simulink model "simulink_interface"  (R2015a)
settings: Solver=ode45  StartTime=0.0  StopTime=inf  RelTol=1e-3
libraries: etargetslib x7, dspbuff3 x3, instrumentlib x3, dspnetwork x3, simulink x1
settings Model: Creator=zev  LastModifiedBy=zev

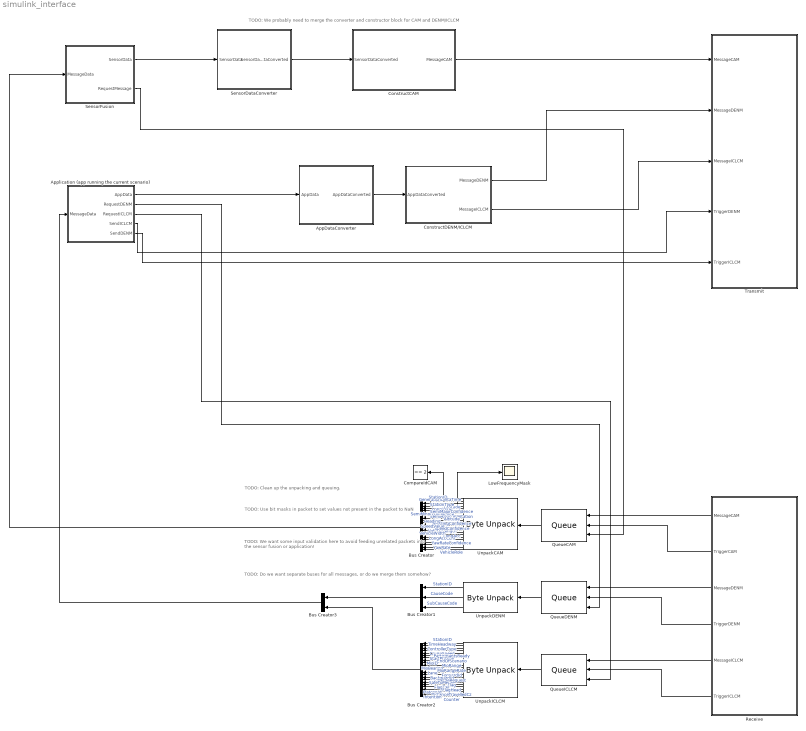
== system simulink_interface ==
  note: TODO: Clean up the unpacking and queuing.
  note: TODO: Do we want separate buses for all messages, or do we merge them somehow?
  note: TODO: Use bit masks in packet to set values not present in the packet to NaN
  note: TODO: We probably need to merge the converter and constructor block for CAM and DENM/ICLCM
  note: TODO: We want some input validation here to avoid feeding unrelated packets
      | into the sensor fusion or application!
  AppDataConverter : Subsystem
  Application (app running the current scenario) : Subsystem
  Bus Creator : BusCreator  Inputs=20
  Bus Creator1 : BusCreator  Inputs=3
  Bus Creator2 : BusCreator  Inputs=23
  Bus Creator3 : BusCreator  Inputs=2
  CompareIdCAM : simulink/Logic and Bit Operations/Compare To Constant  relop===  const=2  OutDataTypeStr=uint8
  ConstructCAM : Subsystem
  ConstructDENM/ICLCM : Subsystem
  LowFrequencyMask : Scope
  QueueCAM : dspbuff3/Queue  depth=8  trigger=Rising edge  overflow=Dynamic reallocation  pes=Warning  eso=off  fso=off  nso=off  clr=off  clrOutport=off  adf=on
  QueueDENM : dspbuff3/Queue  depth=8  trigger=Rising edge  overflow=Dynamic reallocation  pes=Warning  eso=off  fso=off  nso=off  clr=off  clrOutport=off  adf=on
  QueueICLCM : dspbuff3/Queue  depth=8  trigger=Rising edge  overflow=Dynamic reallocation  pes=Warning  eso=off  fso=off  nso=off  clr=off  clrOutport=off  adf=on
  Receive : Subsystem
  SensorDataConverter : Subsystem
  SensorFusion : Subsystem
  Transmit : Subsystem
  UnpackCAM : etargetslib/Byte Unpack  dimensions={[1],[1],[1],[1],[1],[1],[1],[1],[1],[1],[1],[1],[1],[1],[1],[1],[1],[1],[1],[1],[1],[1],}  datatypes={'uint8','int32', 'int32','uint8','int32', 'int32','int32', 'int32','int32', 'int32','int32', 'int32','int32', 'int32','int32', 'int32','int32', 'int32','int32', 'int32','int32', 'int32',}  byteAlign=1
  UnpackDENM : etargetslib/Byte Unpack  dimensions={[1], [1], [1]}  datatypes={'int32', 'int32', 'int32'}  byteAlign=1
  UnpackICLCM : etargetslib/Byte Unpack  dimensions={[1],[1], [1],[1], [1],[1], [1],[1], [1],[1], [1],[1], [1],[1], [1],[1], [1],[1],[1],[1], [1],[1], [1]}  datatypes={'int32','int32', 'int32','int32', 'int32','int32', 'int32','int32', 'int32','int32', 'int32','int32', 'int32','int32', 'int32','int32', 'int32','int32', 'int32','int32', 'int32','int32', 'int32'}  byteAlign=1
  wires:
  UnpackCAM/1 -> CompareIdCAM/1
  UnpackCAM/4 -> LowFrequencyMask/1
  UnpackCAM/22 -> Bus Creator/20  "VehicleRole"
  UnpackCAM/21 -> Bus Creator/19  "YawRateConfidence"
  UnpackCAM/20 -> Bus Creator/18  "YawRate"
  UnpackCAM/19 -> Bus Creator/17  "LongAccConf"
  UnpackCAM/18 -> Bus Creator/16  "LongAcc"
  UnpackCAM/16 -> Bus Creator/14  "VehicleLength"
  UnpackCAM/17 -> Bus Creator/15  "VehicleWidth"
  UnpackCAM/15 -> Bus Creator/13  "SpeedConfidence"
  UnpackCAM/13 -> Bus Creator/11  "HeadingConfidence"
  UnpackCAM/14 -> Bus Creator/12  "SpeedValue"
  UnpackCAM/12 -> Bus Creator/10  "Heading"
  UnpackCAM/10 -> Bus Creator/8  "SemiMajorOrientation"
  UnpackCAM/11 -> Bus Creator/9  "Altitude"
  UnpackCAM/9 -> Bus Creator/7  "SemiMinorConfidence"
  UnpackCAM/7 -> Bus Creator/5  "Longitude"
  UnpackCAM/8 -> Bus Creator/6  "SemiMajorConfidence"
  UnpackCAM/6 -> Bus Creator/4  "Latitude"
  UnpackCAM/5 -> Bus Creator/3  "StationType"
  UnpackCAM/3 -> Bus Creator/2  "GenerationDeltaTime"
  UnpackCAM/2 -> Bus Creator/1  "StationID"
  Bus Creator/1 -> SensorFusion/1(MessageData)
  SensorFusion/2(RequestMessage) -> QueueCAM/3
  QueueCAM/1 -> UnpackCAM/1
  Application (app running the current scenario)/2(RequestDENM) -> QueueDENM/3
  Application (app running the current scenario)/3(RequestICLCM) -> QueueICLCM/3
  QueueDENM/1 -> UnpackDENM/1
  QueueICLCM/1 -> UnpackICLCM/1
  Application (app running the current scenario)/1(AppData) -> AppDataConverter/1(AppData)
  AppDataConverter/1(AppDataConverted) -> ConstructDENM/ICLCM/1(AppDataConverted)
  SensorFusion/1(SensorData) -> SensorDataConverter/1(SensorData)
  SensorDataConverter/1(SensorDataConverted) -> ConstructCAM/1(SensorDataConverted)
  UnpackICLCM/1 -> Bus Creator2/1  "StationID"
  UnpackICLCM/2 -> Bus Creator2/2  "ControllerType"
  UnpackICLCM/3 -> Bus Creator2/3  "TimeHeadway"
  UnpackICLCM/4 -> Bus Creator2/4  "CruiseSpeed"
  UnpackICLCM/5 -> Bus Creator2/5  "ParticipantsReady"
  UnpackICLCM/6 -> Bus Creator2/6  "StartPlatoon"
  UnpackICLCM/7 -> Bus Creator2/7  "EndOfScenario"
  UnpackICLCM/8 -> Bus Creator2/8  "MioID"
  UnpackICLCM/9 -> Bus Creator2/9  "MioRange"
  UnpackICLCM/10 -> Bus Creator2/10  "MioBearing"
  UnpackICLCM/11 -> Bus Creator2/11  "MioRangeRate"
  UnpackICLCM/12 -> Bus Creator2/12  "Lane"
  UnpackICLCM/13 -> Bus Creator2/13  "ForwardId"
  UnpackICLCM/14 -> Bus Creator2/14  "BackwardId"
  UnpackICLCM/15 -> Bus Creator2/15  "MergeRequest"
  UnpackICLCM/16 -> Bus Creator2/16  "SafeToMerge"
  UnpackICLCM/17 -> Bus Creator2/17  "Flag"
  UnpackICLCM/18 -> Bus Creator2/18  "FlagTail"
  UnpackICLCM/19 -> Bus Creator2/19  "FlagHead"
  UnpackICLCM/20 -> Bus Creator2/20  "PlatoonId"
  UnpackICLCM/21 -> Bus Creator2/21  "DistanceTravelledCz"
  UnpackICLCM/22 -> Bus Creator2/22  "Intention"
  Bus Creator1/1 -> Bus Creator3/1
  Bus Creator2/1 -> Bus Creator3/2
  UnpackICLCM/23 -> Bus Creator2/23  "Counter"
  UnpackDENM/1 -> Bus Creator1/1  "StationID"
  UnpackDENM/2 -> Bus Creator1/2  "CauseCode"
  UnpackDENM/3 -> Bus Creator1/3  "SubCauseCode"
  Bus Creator3/1 -> Application (app running the current scenario)/1(MessageData)
  ConstructCAM/1(MessageCAM) -> Transmit/1(MessageCAM)
  ConstructDENM/ICLCM/1(MessageDENM) -> Transmit/2(MessageDENM)
  ConstructDENM/ICLCM/2(MessageICLCM) -> Transmit/3(MessageICLCM)
  Application (app running the current scenario)/4(SendICLCM) -> Transmit/4(TriggerDENM)
  Application (app running the current scenario)/5(SendDENM) -> Transmit/5(TriggerICLCM)
  Receive/1(MessageCAM) -> QueueCAM/1
  Receive/2(TriggerCAM) -> QueueCAM/2
  Receive/3(MessageDENM) -> QueueDENM/1
  Receive/4(TriggerDENM) -> QueueDENM/2
  Receive/5(MessageICLCM) -> QueueICLCM/1
  Receive/6(TriggerICLCM) -> QueueICLCM/2

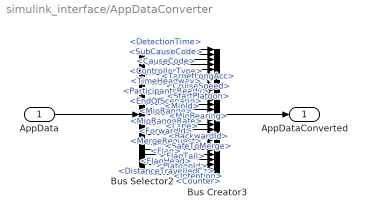
== system simulink_interface/AppDataConverter ==
  AppData : Inport
  Bus Creator3 : BusCreator  Inputs=26
  Bus Selector2 : BusSelector  OutputSignals=DetectionTime,CauseCode,SubCauseCode,ControllerType,TargetLongAcc,TimeHeadway,CruiseSpeed,ParticipantsReady,StartPlatoon,EndOfScenario,MioId,MioRange,MioBearing,MioRangeRate,Lane,ForwardId,BackwardId,MergeRequest,SafeToMerge,Flag,FlagTail,FlagHead,PlatoonId,DistanceTravelledCz,Intention,Counter
  AppDataConverted : Outport
  wires:
  Bus Creator3/1 -> AppDataConverted/1
  AppData/1 -> Bus Selector2/1
  Bus Selector2/1 -> Bus Creator3/1  "<DetectionTime>"
  Bus Selector2/2 -> Bus Creator3/2  "<CauseCode>"
  Bus Selector2/3 -> Bus Creator3/3  "<SubCauseCode>"
  Bus Selector2/4 -> Bus Creator3/4  "<ControllerType>"
  Bus Selector2/5 -> Bus Creator3/5  "<TargetLongAcc>"
  Bus Selector2/6 -> Bus Creator3/6  "<TimeHeadway>"
  Bus Selector2/7 -> Bus Creator3/7  "<CruiseSpeed>"
  Bus Selector2/8 -> Bus Creator3/8  "<ParticipantsReady>"
  Bus Selector2/9 -> Bus Creator3/9  "<StartPlatoon>"
  Bus Selector2/10 -> Bus Creator3/10  "<EndOfScenario>"
  Bus Selector2/11 -> Bus Creator3/11  "<MioId>"
  Bus Selector2/12 -> Bus Creator3/12  "<MioRange>"
  Bus Selector2/13 -> Bus Creator3/13  "<MioBearing>"
  Bus Selector2/14 -> Bus Creator3/14  "<MioRangeRate>"
  Bus Selector2/15 -> Bus Creator3/15  "<Lane>"
  Bus Selector2/16 -> Bus Creator3/16  "<ForwardId>"
  Bus Selector2/17 -> Bus Creator3/17  "<BackwardId>"
  Bus Selector2/18 -> Bus Creator3/18  "<MergeRequest>"
  Bus Selector2/19 -> Bus Creator3/19  "<SafeToMerge>"
  Bus Selector2/20 -> Bus Creator3/20  "<Flag>"
  Bus Selector2/21 -> Bus Creator3/21  "<FlagTail>"
  Bus Selector2/22 -> Bus Creator3/22  "<FlagHead>"
  Bus Selector2/23 -> Bus Creator3/23  "<PlatoonId>"
  Bus Selector2/24 -> Bus Creator3/24  "<DistanceTravelledCz>"
  Bus Selector2/25 -> Bus Creator3/25  "<Intention>"
  Bus Selector2/26 -> Bus Creator3/26  "<Counter>"

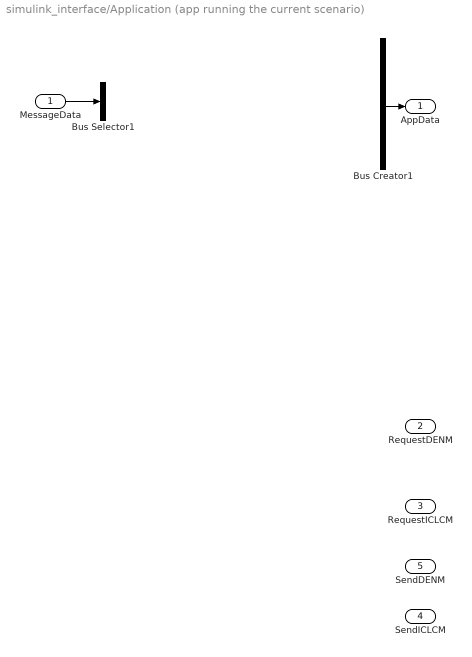
== system simulink_interface/Application (app running the current scenario) ==
  MessageData : Inport
  Bus Creator1 : BusCreator  Inputs=26
  Bus Selector1 : BusSelector  OutputSignals=signal1,signal2
  AppData : Outport
  RequestDENM : Outport  Port=2
  RequestICLCM : Outport  Port=3
  SendICLCM : Outport  Port=4
  SendDENM : Outport  Port=5
  wires:
  MessageData/1 -> Bus Selector1/1
  Bus Creator1/1 -> AppData/1
  ? -> Bus Creator1/1  "DetectionTime"
  ? -> Bus Creator1/2  "CauseCode"
  ? -> Bus Creator1/3  "SubCauseCode"
  ? -> Bus Creator1/4  "ControllerType"
  ? -> Bus Creator1/5  "TargetLongAcc"
  ? -> Bus Creator1/6  "TimeHeadway"
  ? -> Bus Creator1/7  "CruiseSpeed"
  ? -> Bus Creator1/8  "ParticipantsReady"
  ? -> Bus Creator1/9  "StartPlatoon"
  ? -> Bus Creator1/10  "EndOfScenario"
  ? -> Bus Creator1/11  "MioId"
  ? -> Bus Creator1/12  "MioRange"
  ? -> Bus Creator1/13  "MioBearing"
  ? -> Bus Creator1/14  "MioRangeRate"
  ? -> Bus Creator1/15  "Lane"
  ? -> Bus Creator1/16  "ForwardId"
  ? -> Bus Creator1/17  "BackwardId"
  ? -> Bus Creator1/18  "MergeRequest"
  ? -> Bus Creator1/19  "SafeToMerge"
  ? -> Bus Creator1/20  "Flag"
  ? -> Bus Creator1/21  "FlagTail"
  ? -> Bus Creator1/22  "FlagHead"
  ? -> Bus Creator1/23  "PlatoonId"
  ? -> Bus Creator1/24  "DistanceTravelledCz"
  ? -> Bus Creator1/25  "Intention"
  ? -> Bus Creator1/26  "Counter"

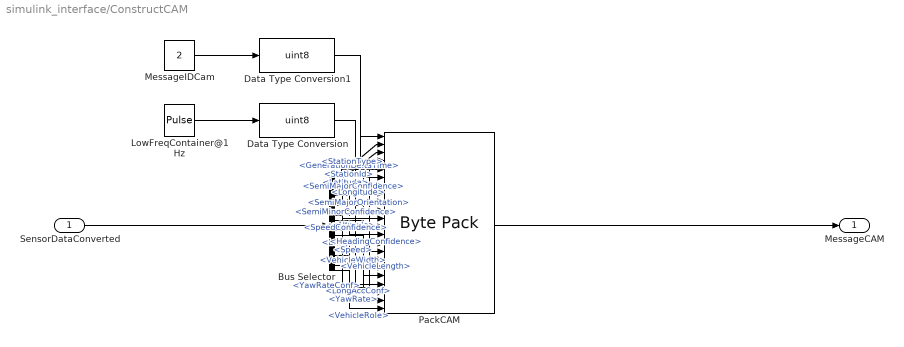
== system simulink_interface/ConstructCAM ==
  SensorDataConverted : Inport
  Bus Selector : BusSelector  OutputSignals=StationId,GenerationDeltaTime,StationType,Latitude,Longitude,SemiMajorConfidence,SemiMinorConfidence,SemiMajorOrientation,Altitude,Heading,HeadingConfidence,Speed,SpeedConfidence,VehicleLength,VehicleWidth,LongAcc,LongAccConf,YawRate,YawRateConf,VehicleRole
  Data Type Conversion : DataTypeConversion  OutDataTypeStr=uint8
  Data Type Conversion1 : DataTypeConversion  OutDataTypeStr=uint8
  LowFreqContainer@1Hz : DiscretePulseGenerator  PulseType=Time based  Amplitude=128  Period=1  PulseWidth=0.04
  MessageIDCam : Constant  Value=2
  PackCAM : etargetslib/Byte Pack  datatypes={'uint8','int32', 'int32','uint8','int32', 'int32','int32', 'int32','int32', 'int32','int32', 'int32','int32', 'int32','int32', 'int32','int32', 'int32','int32', 'int32','int32', 'int32',}  byteAlign=1
  MessageCAM : Outport
  wires:
  Bus Selector/8 -> PackCAM/10  "<SemiMajorOrientation>"
  Bus Selector/4 -> PackCAM/6  "<Latitude>"
  Bus Selector/2 -> PackCAM/3  "<GenerationDeltaTime>"
  Bus Selector/9 -> PackCAM/11  "<Altitude>"
  Bus Selector/6 -> PackCAM/8  "<SemiMajorConfidence>"
  Bus Selector/7 -> PackCAM/9  "<SemiMinorConfidence>"
  Bus Selector/1 -> PackCAM/2  "<StationId>"
  PackCAM/1 -> MessageCAM/1
  Bus Selector/3 -> PackCAM/5  "<StationType>"
  Data Type Conversion/1 -> PackCAM/4
  MessageIDCam/1 -> Data Type Conversion1/1
  Bus Selector/5 -> PackCAM/7  "<Longitude>"
  Bus Selector/15 -> PackCAM/17  "<VehicleWidth>"
  Bus Selector/10 -> PackCAM/12  "<Heading>"
  Bus Selector/16 -> PackCAM/18  "<LongAcc>"
  Bus Selector/12 -> PackCAM/14  "<Speed>"
  Bus Selector/17 -> PackCAM/19  "<LongAccConf>"
  Bus Selector/11 -> PackCAM/13  "<HeadingConfidence>"
  Bus Selector/14 -> PackCAM/16  "<VehicleLength>"
  Bus Selector/13 -> PackCAM/15  "<SpeedConfidence>"
  SensorDataConverted/1 -> Bus Selector/1
  Data Type Conversion1/1 -> PackCAM/1
  Bus Selector/19 -> PackCAM/21  "<YawRateConf>"
  Bus Selector/20 -> PackCAM/22  "<VehicleRole>"
  LowFreqContainer@1Hz/1 -> Data Type Conversion/1
  Bus Selector/18 -> PackCAM/20  "<YawRate>"

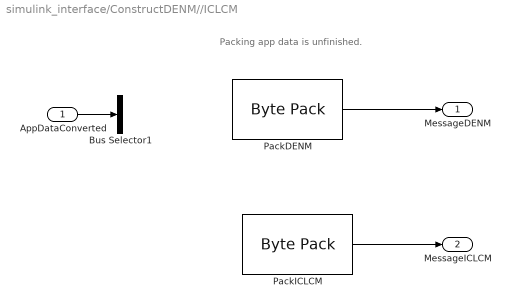
== system simulink_interface/ConstructDENM//ICLCM ==
  note: Packing app data is unfinished.
  AppDataConverted : Inport
  Bus Selector1 : BusSelector  OutputSignals=signal1,signal2
  PackDENM : etargetslib/Byte Pack  datatypes={'int32', 'int32'}  byteAlign=1
  PackICLCM : etargetslib/Byte Pack  datatypes={'int32', 'int32'}  byteAlign=1
  MessageDENM : Outport
  MessageICLCM : Outport  Port=2
  wires:
  PackDENM/1 -> MessageDENM/1
  AppDataConverted/1 -> Bus Selector1/1
  PackICLCM/1 -> MessageICLCM/1

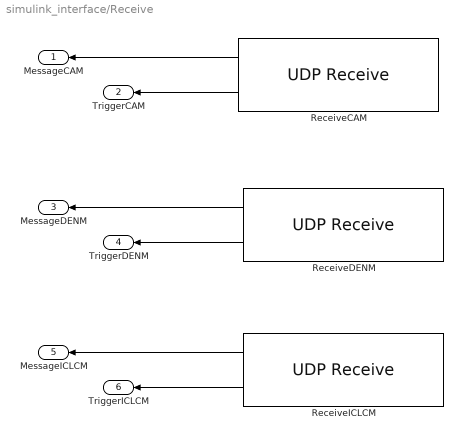
== system simulink_interface/Receive ==
  ReceiveCAM : instrumentlib/UDP Receive  Host=0.0.0.0  Port=5000  LocalPort=-1  DataSize="[1  82]"  EnableBlockingMode=off  Timeout=10  SampleTime=0.01  DataType=uint8  ByteOrder=BigEndian
  ReceiveDENM : instrumentlib/UDP Receive  Host=0.0.0.0  Port=5000  LocalPort=-1  DataSize="[1  82]"  EnableBlockingMode=off  Timeout=10  SampleTime=0.01  DataType=uint8  ByteOrder=BigEndian
  ReceiveICLCM : instrumentlib/UDP Receive  Host=0.0.0.0  Port=5000  LocalPort=-1  DataSize="[1  82]"  EnableBlockingMode=off  Timeout=10  SampleTime=0.01  DataType=uint8  ByteOrder=BigEndian
  MessageCAM : Outport
  TriggerCAM : Outport  Port=2
  MessageDENM : Outport  Port=3
  TriggerDENM : Outport  Port=4
  MessageICLCM : Outport  Port=5
  TriggerICLCM : Outport  Port=6
  wires:
  ReceiveCAM/1 -> MessageCAM/1
  ReceiveICLCM/2 -> TriggerICLCM/1
  ReceiveICLCM/1 -> MessageICLCM/1
  ReceiveDENM/2 -> TriggerDENM/1
  ReceiveDENM/1 -> MessageDENM/1
  ReceiveCAM/2 -> TriggerCAM/1

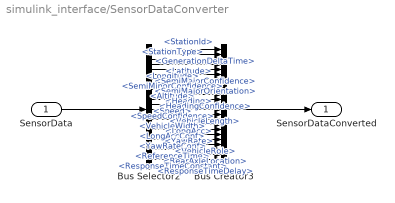
== system simulink_interface/SensorDataConverter ==
  SensorData : Inport
  Bus Creator3 : BusCreator  Inputs=24
  Bus Selector2 : BusSelector  OutputSignals=StationId,GenerationDeltaTime,StationType,Latitude,Longitude,SemiMajorConfidence,SemiMinorConfidence,SemiMajorOrientation,Altitude,Heading,HeadingConfidence,Speed,SpeedConfidence,VehicleLength,VehicleWidth,LongAcc,LongAccConf,YawRate,YawRateConf,VehicleRole,ReferenceTime,RearAxleLocation,ResponseTimeConstant,ResponseTimeDelay
  SensorDataConverted : Outport
  wires:
  Bus Creator3/1 -> SensorDataConverted/1
  SensorData/1 -> Bus Selector2/1
  Bus Selector2/1 -> Bus Creator3/1  "<StationId>"
  Bus Selector2/2 -> Bus Creator3/2  "<GenerationDeltaTime>"
  Bus Selector2/3 -> Bus Creator3/3  "<StationType>"
  Bus Selector2/4 -> Bus Creator3/4  "<Latitude>"
  Bus Selector2/5 -> Bus Creator3/5  "<Longitude>"
  Bus Selector2/6 -> Bus Creator3/6  "<SemiMajorConfidence>"
  Bus Selector2/7 -> Bus Creator3/7  "<SemiMinorConfidence>"
  Bus Selector2/8 -> Bus Creator3/8  "<SemiMajorOrientation>"
  Bus Selector2/9 -> Bus Creator3/9  "<Altitude>"
  Bus Selector2/10 -> Bus Creator3/10  "<Heading>"
  Bus Selector2/11 -> Bus Creator3/11  "<HeadingConfidence>"
  Bus Selector2/12 -> Bus Creator3/12  "<Speed>"
  Bus Selector2/13 -> Bus Creator3/13  "<SpeedConfidence>"
  Bus Selector2/14 -> Bus Creator3/14  "<VehicleLength>"
  Bus Selector2/15 -> Bus Creator3/15  "<VehicleWidth>"
  Bus Selector2/16 -> Bus Creator3/16  "<LongAcc>"
  Bus Selector2/17 -> Bus Creator3/17  "<LongAccConf>"
  Bus Selector2/18 -> Bus Creator3/18  "<YawRate>"
  Bus Selector2/19 -> Bus Creator3/19  "<YawRateConf>"
  Bus Selector2/20 -> Bus Creator3/20  "<VehicleRole>"
  Bus Selector2/21 -> Bus Creator3/21  "<ReferenceTime>"
  Bus Selector2/22 -> Bus Creator3/22  "<RearAxleLocation>"
  Bus Selector2/23 -> Bus Creator3/23  "<ResponseTimeConstant>"
  Bus Selector2/24 -> Bus Creator3/24  "<ResponseTimeDelay>"

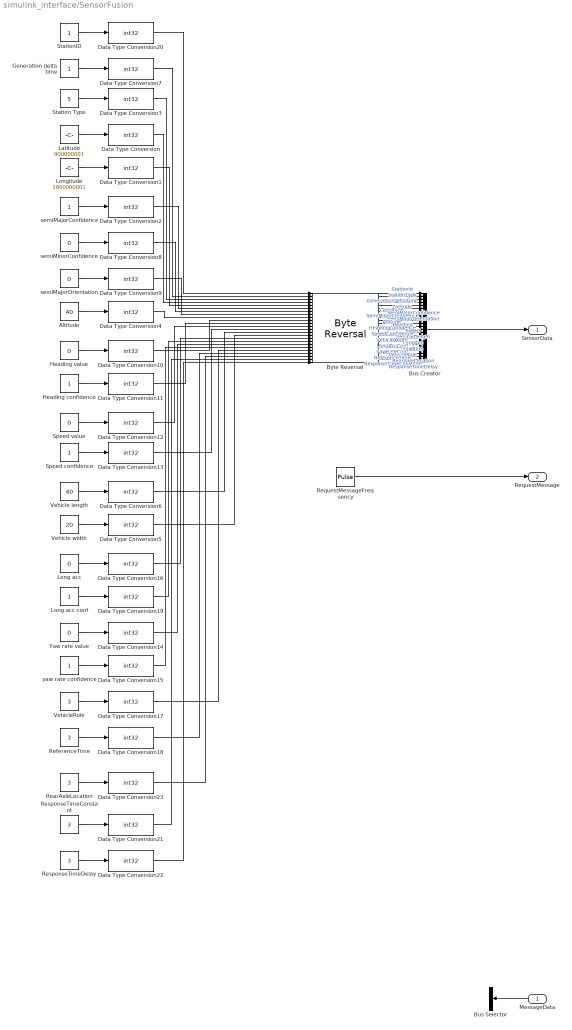
== system simulink_interface/SensorFusion ==
  MessageData : Inport
  Altitude : Constant  Value=40
  Bus Creator : BusCreator  Inputs=24
  Bus Selector : BusSelector  OutputSignals=StationID,GenerationDeltaTime
  Byte Reversal : etargetslib/Byte Reversal  numInp=24
  Data Type Conversion{,1..23} (24 alike) : DataTypeConversion  OutDataTypeStr=int32
  Generation delta time : Constant
  Heading confidence : Constant
  Heading value : Constant  Value=0
  Latitude : Constant  Value=900000001
  Long acc : Constant  Value=0
  Long acc conf : Constant
  Longitude : Constant  Value=1800000001
  RearAxleLocation : Constant  Value=3
  ReferenceTime : Constant  Value=3
  RequestMessageFrequency : DiscretePulseGenerator  PulseType=Time based  Period=0.01  PulseWidth=5
  ResponseTimeConstant : Constant  Value=3
  ResponseTimeDelay : Constant  Value=3
  Speed confidence : Constant
  Speed value : Constant  Value=0
  Station Type : Constant  Value=5
  StationID : Constant
  Vehicle length : Constant  Value=40
  Vehicle width : Constant  Value=20
  VehicleRole : Constant  Value=3
  Yaw rate value : Constant  Value=0
  "semiMajorConfidence " : Constant
  "semiMajorOrientation " : Constant  Value=0
  "semiMinorConfidence " : Constant  Value=0
  yaw rate confidence : Constant
  SensorData : Outport
  RequestMessage : Outport  Port=2
  wires:
  Bus Creator/1 -> SensorData/1
  Station Type/1 -> Data Type Conversion3/1
  Generation delta time/1 -> Data Type Conversion7/1
  yaw rate confidence/1 -> Data Type Conversion15/1
  Long acc/1 -> Data Type Conversion16/1
  VehicleRole/1 -> Data Type Conversion17/1
  Long acc conf/1 -> Data Type Conversion19/1
  ReferenceTime/1 -> Data Type Conversion18/1
  Vehicle length/1 -> Data Type Conversion6/1
  Vehicle width/1 -> Data Type Conversion5/1
  Latitude/1 -> Data Type Conversion/1
  Longitude/1 -> Data Type Conversion1/1
  "semiMajorConfidence "/1 -> Data Type Conversion2/1
  "semiMinorConfidence "/1 -> Data Type Conversion8/1
  "semiMajorOrientation "/1 -> Data Type Conversion9/1
  Heading confidence/1 -> Data Type Conversion11/1
  Heading value/1 -> Data Type Conversion10/1
  Speed value/1 -> Data Type Conversion12/1
  Speed confidence/1 -> Data Type Conversion13/1
  Yaw rate value/1 -> Data Type Conversion14/1
  StationID/1 -> Data Type Conversion20/1
  Altitude/1 -> Data Type Conversion4/1
  ResponseTimeConstant/1 -> Data Type Conversion21/1
  ResponseTimeDelay/1 -> Data Type Conversion22/1
  RearAxleLocation/1 -> Data Type Conversion23/1
  Data Type Conversion20/1 -> Byte Reversal/1
  Data Type Conversion7/1 -> Byte Reversal/2
  Data Type Conversion3/1 -> Byte Reversal/3
  Data Type Conversion/1 -> Byte Reversal/4
  Data Type Conversion1/1 -> Byte Reversal/5
  Data Type Conversion2/1 -> Byte Reversal/6
  Data Type Conversion8/1 -> Byte Reversal/7
  Data Type Conversion9/1 -> Byte Reversal/8
  Data Type Conversion4/1 -> Byte Reversal/9
  Data Type Conversion10/1 -> Byte Reversal/10
  Data Type Conversion11/1 -> Byte Reversal/11
  Data Type Conversion12/1 -> Byte Reversal/12
  Data Type Conversion13/1 -> Byte Reversal/13
  Data Type Conversion6/1 -> Byte Reversal/14
  Data Type Conversion5/1 -> Byte Reversal/15
  Data Type Conversion16/1 -> Byte Reversal/16
  Data Type Conversion19/1 -> Byte Reversal/17
  Data Type Conversion14/1 -> Byte Reversal/18
  Data Type Conversion15/1 -> Byte Reversal/19
  Data Type Conversion17/1 -> Byte Reversal/20
  Data Type Conversion18/1 -> Byte Reversal/21
  Data Type Conversion23/1 -> Byte Reversal/22
  Data Type Conversion21/1 -> Byte Reversal/23
  Data Type Conversion22/1 -> Byte Reversal/24
  Byte Reversal/1 -> Bus Creator/1  "StationId"
  Byte Reversal/2 -> Bus Creator/2  "GenerationDeltaTime"
  Byte Reversal/3 -> Bus Creator/3  "StationType"
  Byte Reversal/4 -> Bus Creator/4  "Latitude"
  Byte Reversal/5 -> Bus Creator/5  "Longitude"
  Byte Reversal/6 -> Bus Creator/6  "SemiMajorConfidence"
  Byte Reversal/7 -> Bus Creator/7  "SemiMinorConfidence"
  Byte Reversal/8 -> Bus Creator/8  "SemiMajorOrientation"
  Byte Reversal/9 -> Bus Creator/9  "Altitude"
  Byte Reversal/10 -> Bus Creator/10  "Heading"
  Byte Reversal/11 -> Bus Creator/11  "HeadingConfidence"
  Byte Reversal/12 -> Bus Creator/12  "Speed"
  Byte Reversal/13 -> Bus Creator/13  "SpeedConfidence"
  Byte Reversal/14 -> Bus Creator/14  "VehicleLength"
  Byte Reversal/15 -> Bus Creator/15  "VehicleWidth"
  Byte Reversal/16 -> Bus Creator/16  "LongAcc"
  Byte Reversal/17 -> Bus Creator/17  "LongAccConf"
  Byte Reversal/18 -> Bus Creator/18  "YawRate"
  Byte Reversal/19 -> Bus Creator/19  "YawRateConf"
  Byte Reversal/20 -> Bus Creator/20  "VehicleRole"
  Byte Reversal/21 -> Bus Creator/21  "ReferenceTime"
  Byte Reversal/22 -> Bus Creator/22  "RearAxleLocation"
  Byte Reversal/23 -> Bus Creator/23  "ResponseTimeConstant"
  Byte Reversal/24 -> Bus Creator/24  "ResponseTimeDelay"
  RequestMessageFrequency/1 -> RequestMessage/1
  MessageData/1 -> Bus Selector/1

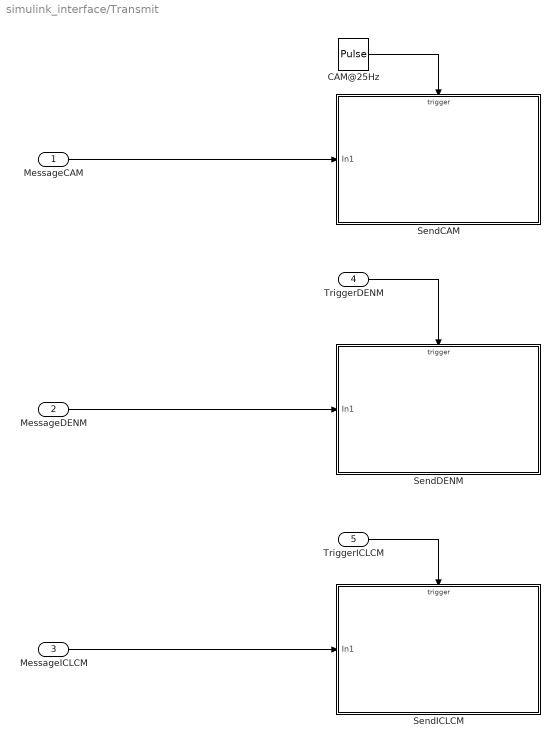
== system simulink_interface/Transmit ==
  MessageCAM : Inport
  MessageDENM : Inport  Port=2
  MessageICLCM : Inport  Port=3
  TriggerDENM : Inport  Port=4
  TriggerICLCM : Inport  Port=5
  CAM@25Hz : DiscretePulseGenerator  PulseType=Time based  Period=0.04  PulseWidth=5
  SendCAM : Subsystem
  SendDENM : Subsystem
  SendICLCM : Subsystem
  wires:
  MessageDENM/1 -> SendDENM/1(In1)
  MessageICLCM/1 -> SendICLCM/1(In1)
  TriggerDENM/1 -> SendDENM/Trigger
  TriggerICLCM/1 -> SendICLCM/Trigger
  CAM@25Hz/1 -> SendCAM/Trigger
  MessageCAM/1 -> SendCAM/1(In1)

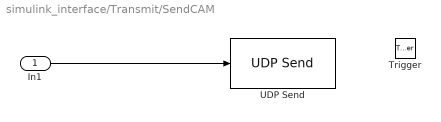
== system simulink_interface/Transmit/SendCAM ==
  In1 : Inport
  Trigger : TriggerPort  PortDimensions=1
  UDP Send : dspnetwork/UDP Send  remoteURL='127.0.0.1'  remotePort=5001  localURL='0.0.0.0'  localPortSource=Automatically determine  localPort=-1  sampletime=-1  separateLengthPort=0
  wires:
  In1/1 -> UDP Send/1

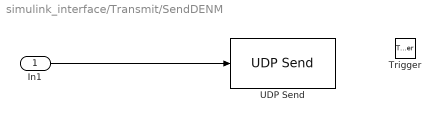
== system simulink_interface/Transmit/SendDENM ==
  In1 : Inport
  Trigger : TriggerPort  PortDimensions=1
  UDP Send : dspnetwork/UDP Send  remoteURL='127.0.0.1'  remotePort=5001  localURL='0.0.0.0'  localPortSource=Automatically determine  localPort=-1  sampletime=-1  separateLengthPort=0
  wires:
  In1/1 -> UDP Send/1

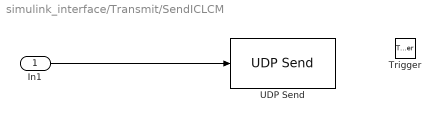
== system simulink_interface/Transmit/SendICLCM ==
  In1 : Inport
  Trigger : TriggerPort  PortDimensions=1
  UDP Send : dspnetwork/UDP Send  remoteURL='127.0.0.1'  remotePort=5001  localURL='0.0.0.0'  localPortSource=Automatically determine  localPort=-1  sampletime=-1  separateLengthPort=0
  wires:
  In1/1 -> UDP Send/1
